simulink model "Copy_of_Robot_PD_Trajectory_Control_"  (R2020b)
settings: Solver=VariableStepAuto  StartTime=0.0  StopTime=6  RelTol=1e-3  EnableMultiTasking=on
model workspace: external: MATLAB File D:\Google Drive\Duongw_Folder\Thesis Master\_Model\Delta_Model_ADEPT\SIMCAPE_MULTI_BODY\ADEPT_DELTA_3AXES1\Assem1_ADEPT_HORNET_DataFile.m (data not in the file)
values from neighbouring files (symbols this model uses):
  G = -5    [Assem1_ADEPT_HORNET_DataFile.m]    (also in data_specMotor.m)
  Kb = 0.4    [Assem1_ADEPT_HORNET_DataFile.m]    (also in data_specMotor.m)
  Km = 0.7    [Assem1_ADEPT_HORNET_DataFile.m]    (also in data_specMotor.m)
  La = 0.0062000000000000006    (= 0.0062)    [Assem1_ADEPT_HORNET_DataFile.m]    (also in data_specMotor.m)
  m = zeros(1,3)    [forward.m]    (also in solequa.m = zeros(3,1))
  Ra = 1.8    [Assem1_ADEPT_HORNET_DataFile.m]    (also in data_specMotor.m)
  smiData = struct    [Assem1_ADEPT_HORNET_DataFile.m]
undefined symbols (not defined in the file or in its folder): X, Y, Z
libraries: sm_lib x106, nesl_utility x7, pid_lib x3
(part 4 of 4)

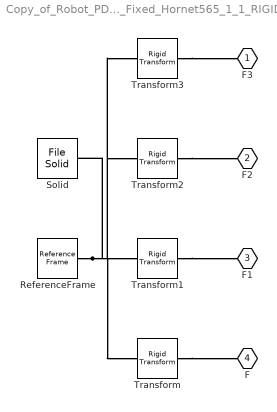
== system Copy_of_Robot_PD_Trajectory_Control_/DELTA ROBOT MODEL/Platform_Fixed_Hornet565_1_1_RIGID ==
  ReferenceFrame : sm_lib/Frames and Transforms/Reference Frame
  Solid : sm_lib/Body Elements/File Solid  ExtGeomFileName=Platform_Fixed-Hornet565_1_Default_sldprt.STEP  UnitType=FromFile  ExtGeomFileUnits=m  StepReaderType=HEX  ExportConvexHullGeometry=off  InertiaType=Custom  Mass=smiData.Solid(5).mass  MassUnits=kg  CenterOfMass=smiData.Solid(5).CoM  CenterOfMassUnits=mm  MomentsOfInertia=smiData.Solid(5).MoI  MomentsOfInertiaUnits=kg*mm^2  ProductsOfInertia=smiData.Solid(5).PoI  ProductsOfInertiaUnits=kg*mm^2  BasedOnType=Density  Density=1000  DensityUnits=kg/(m^3)  DoExposeReferenceFrame=on  SerializedFrames=<Frames/>  GraphicType=FromGeometry  MarkerShape=Sphere  MarkerSize=10  GraphicVisPropType=SimpleVisualProperties  GraphicDiffuseColor=smiData.Solid(5).color  GraphicSpecularColor=[0.5 0.5 0.5 1.0]  GraphicAmbientColor=[0.15 0.15 0.15 1.0]  GraphicEmissiveColor=[0.0 0.0 0.0 1.0]  GraphicShininess=75  GraphicOpacity=smiData.Solid(5).opacity
  Transform : sm_lib/Frames and Transforms/Rigid Transform  TranslationMethod=Cartesian  TranslationStandardOffset=0  TranslationLengthUnit=mm  TranslationStandardAxis=+Z  TranslationCartesianOffset=smiData.RigidTransform(1).translation  TranslationROffset=0  TranslationROffsetUnits=m  TranslationZOffset=0  TranslationZOffsetUnits=m  TranslationThetaOffset=0  TranslationThetaOffsetUnits=deg  RotationMethod=ArbitraryAxis  RotationAngleUnits=rad  RotationStandardAxis=+Z  RotationAngle=smiData.RigidTransform(1).angle  RotationArbitraryAxis=smiData.RigidTransform(1).axis  FollAlignAxisA=+X  BaseAlignAxisA=+Y  FollAlignAxisB=+Y  BaseAlignAxisB=+Z  RotationSequenceAxes=FollowerAxes  RotationSequence=XYX  RotationSequenceAngles=[0 0 0]  RotationSequenceAnglesUnits=deg  RotationMatrix=[1 0 0; 0 1 0; 0 0 1]
  Transform1 : sm_lib/Frames and Transforms/Rigid Transform  TranslationMethod=Cartesian  TranslationStandardOffset=0  TranslationLengthUnit=mm  TranslationStandardAxis=+Z  TranslationCartesianOffset=smiData.RigidTransform(32).translation  TranslationROffset=0  TranslationROffsetUnits=m  TranslationZOffset=0  TranslationZOffsetUnits=m  TranslationThetaOffset=0  TranslationThetaOffsetUnits=deg  RotationMethod=ArbitraryAxis  RotationAngleUnits=rad  RotationStandardAxis=+Z  RotationAngle=smiData.RigidTransform(32).angle  RotationArbitraryAxis=smiData.RigidTransform(32).axis  FollAlignAxisA=+X  BaseAlignAxisA=+Y  FollAlignAxisB=+Y  BaseAlignAxisB=+Z  RotationSequenceAxes=FollowerAxes  RotationSequence=XYX  RotationSequenceAngles=[0 0 0]  RotationSequenceAnglesUnits=deg  RotationMatrix=[1 0 0; 0 1 0; 0 0 1]
  Transform2 : sm_lib/Frames and Transforms/Rigid Transform  TranslationMethod=Cartesian  TranslationStandardOffset=0  TranslationLengthUnit=mm  TranslationStandardAxis=+Z  TranslationCartesianOffset=smiData.RigidTransform(38).translation  TranslationROffset=0  TranslationROffsetUnits=m  TranslationZOffset=0  TranslationZOffsetUnits=m  TranslationThetaOffset=0  TranslationThetaOffsetUnits=deg  RotationMethod=ArbitraryAxis  RotationAngleUnits=rad  RotationStandardAxis=+Z  RotationAngle=smiData.RigidTransform(38).angle  RotationArbitraryAxis=smiData.RigidTransform(38).axis  FollAlignAxisA=+X  BaseAlignAxisA=+Y  FollAlignAxisB=+Y  BaseAlignAxisB=+Z  RotationSequenceAxes=FollowerAxes  RotationSequence=XYX  RotationSequenceAngles=[0 0 0]  RotationSequenceAnglesUnits=deg  RotationMatrix=[1 0 0; 0 1 0; 0 0 1]
  Transform3 : sm_lib/Frames and Transforms/Rigid Transform  TranslationMethod=Cartesian  TranslationStandardOffset=0  TranslationLengthUnit=mm  TranslationStandardAxis=+Z  TranslationCartesianOffset=smiData.RigidTransform(44).translation  TranslationROffset=0  TranslationROffsetUnits=m  TranslationZOffset=0  TranslationZOffsetUnits=m  TranslationThetaOffset=0  TranslationThetaOffsetUnits=deg  RotationMethod=ArbitraryAxis  RotationAngleUnits=rad  RotationStandardAxis=+Z  RotationAngle=smiData.RigidTransform(44).angle  RotationArbitraryAxis=smiData.RigidTransform(44).axis  FollAlignAxisA=+X  BaseAlignAxisA=+Y  FollAlignAxisB=+Y  BaseAlignAxisB=+Z  RotationSequenceAxes=FollowerAxes  RotationSequence=XYX  RotationSequenceAngles=[0 0 0]  RotationSequenceAnglesUnits=deg  RotationMatrix=[1 0 0; 0 1 0; 0 0 1]
  F3 : PMIOPort  Side=Left
  F2 : PMIOPort  Port=2  Side=Left
  F1 : PMIOPort  Port=3  Side=Left
  F : PMIOPort  Port=4  Side=Right
  connections:
  Solid/RConn1 -- ReferenceFrame/RConn1 -- Transform/LConn1 -- Transform1/LConn1 -- Transform2/LConn1 -- Transform3/LConn1
  Transform/RConn1 -- F/RConn1
  Transform1/RConn1 -- F1/RConn1
  Transform2/RConn1 -- F2/RConn1
  Transform3/RConn1 -- F3/RConn1

== matlab function Copy_of_Robot_PD_Trajectory_Control_/MATLAB Function ==
  data: u input; y output
function y = fcn(u)
if(u<1)
    y=0;
else
    y=0.85;
end

== matlab function Copy_of_Robot_PD_Trajectory_Control_/Inverse_Kinematics/MATLAB Function ==
  data: x input; theta1 output; y input; z input; theta2 output; theta3 output
function [theta1, theta2, theta3] = fcn(x,y,z)
%Ham giai bai toan dong hoc nguoc
%phuong trinh dong hoc nguoc : a*cos(theta)+b*sin(theta) = c
r1 = 0.225; % Radius of circle crosses three revolute joints of the Base
r2 = 0.075;  % Radius of circle crosses three revolute joints of the Moving platform
r = r2 - r1;
l1 = 0.315;         % Kinematics Length of Active arms
l2 = 0.825;         % Kinematics length of Driven arms
phi1 = pi/2;
phi2 = 7*pi/6;
phi3 = 11*pi/6;
phi = [phi1; phi2; phi3];
%--------------------------------------------------------------------------
    a1 = 2*l1*(r+x*cos(phi(1))+y*sin(phi(1)));
    b1 = 2*z*l1;
    c1 = x^2 + y^2 + z^2 + r^2 +l1^2-l2^2+2*r*(y*sin(phi(1))+x*cos(phi(1)));
    anfa1 = asin(a1/(sqrt(a1^2+b1^2)));
    theta1 = asin(c1/(sqrt(a1^2+b1^2)))- anfa1;
%--------------------------------------------------------------------------
    a2 = 2*l1*(r+x*cos(phi(2))+y*sin(phi(2)));
    b2 = 2*z*l1;
    c2 = x^2 + y^2 + z^2 + r^2 +l1^2-l2^2+2*r*(y*sin(phi(2))+x*cos(phi(2)));
    anfa2 = asin(a2/(sqrt(a2^2+b2^2)));
    theta2 = asin(c2/(sqrt(a2^2+b2^2)))- anfa2;
%--------------------------------------------------------------------------
    a3 = 2*l1*(r+x*cos(phi(3))+y*sin(phi(3)));
    b3 = 2*z*l1;
    c3 = x^2 + y^2 + z^2 + r^2 +l1^2-l2^2+2*r*(y*sin(phi(3))+x*cos(phi(3)));
    anfa3 = asin(a3/(sqrt(a3^2+b3^2)));
    theta3 = asin(c3/(sqrt(a3^2+b3^2)))- anfa3;

== matlab function Copy_of_Robot_PD_Trajectory_Control_/MATLAB Function1 ==
  data: u1 input; y output; u2 input
function y = fcn(u1, u2)

y = u2/u1;

== matlab function Copy_of_Robot_PD_Trajectory_Control_/MATLAB Function2 ==
  data: u1 input; y output; u2 input
function y = fcn(u1, u2)

y = u2/u1;
